simulink model "DF001A_FltInj"  (R2013b)
settings: Solver=FixedStepDiscrete  StartTime=0.0  StopTime=1  FixedStep=.002  RelTol=1e-3
values from neighbouring files (symbols this model uses):
  ARCHGLBPRM_180OVERPI_ULS_F32 = DataDict.Constant    [DF001A_FltInj_DataDict.m]
  ARCHGLBPRM_2PI_ULS_F32 = DataDict.Constant    [DF001A_FltInj_DataDict.m]
  FLOATTOU0P16MULT_ULS_F32 = DataDict.Constant    [DF001A_FltInj_DataDict.m]
  TICNVN_MILLISECPERCNT_F32 = DataDict.Constant    [DF001A_FltInj_DataDict.m]
libraries: simulink x6, NxtrLim x2, NxtrAbslt x1, NxtrMath x1, FixdToFloat x1
(part 2 of 2)

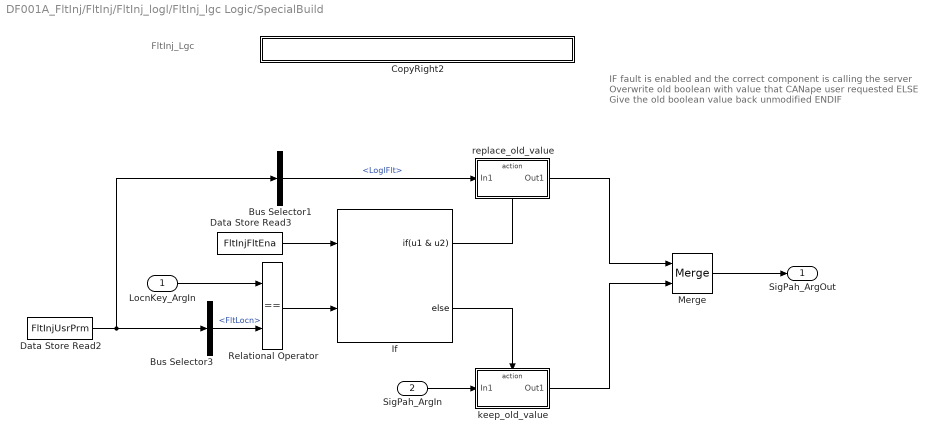
== system DF001A_FltInj/FltInj/FltInj_logl/FltInj_lgc Logic/SpecialBuild ==
  note: IF  fault is enabled and the correct component is calling the server
      |     Overwrite old boolean with value that CANape user requested
      | ELSE
      |     Give the old boolean value back unmodified
      | ENDIF
  note: FltInj_Lgc
  LocnKey_ArgIn : Inport  RequirementInfo={} %GIDa_ad100357_96bd_46c3_ad57_bbc8d7f94a2d
  SigPah_ArgIn : Inport  RequirementInfo={} %GIDa_10444aa2_7cb6_4718_9162_edb39688d745  Port=2
  Bus Selector1 : BusSelector  OutputSignals=LoglFlt
  Bus Selector3 : BusSelector  OutputSignals=FltLocn
  CopyRight2 : Subsystem  Description=|  mask(Copyright Information){none=on}
      | Copyright info block.                                               
      |                                                                     
      | Place copyright information at the top of every subsystem in design.
      mask prompts: none "No parameters"
      mask help: Place copyright information at the top of every subsystem in design.
      mask Display:
      | NxtrConf = 'Nexteer Confidential';
      | 
      | sys = bdroot; %handle for the current model ("system")
      | first = get_param(sys,'Created');
      | if(isempty(first))
      |     first = datestr(now,'yyyy');
      | else
      |     first = first(end-3:end);  %year is last four digits
      | end
      | 
      | last = get_param(sys,'LastModifiedDate');
      | if isempty(last)
      |     last = datestr(now,'yyyy');
      | else
      |     last = last(end-3:end);
      | end
      | 
      | if strcmp(first,last)
      |     fprintf('%s -- Copyright %s Nexteer',NxtrConf,first)
      | else
      |     fprintf('%s -- %s%s- %s Nexteer',NxtrConf,char(169),first,last)
      | end
  Data Store Read2 : DataStoreRead  DataStoreName=FltInjUsrPrm
  Data Store Read3 : DataStoreRead  DataStoreName=FltInjFltEna
  If : If  NumInputs=2  IfExpression=u1 & u2
  Merge : Merge
  Relational Operator : RelationalOperator  Operator===
  keep_old_value : Subsystem  TreatAsAtomicUnit=on
  replace_old_value : Subsystem  TreatAsAtomicUnit=on
  SigPah_ArgOut : Outport
  wires:
  Merge/1 -> SigPah_ArgOut/1
  Data Store Read2/1 -> Bus Selector1/1, Bus Selector3/1
  Bus Selector3/1 -> Relational Operator/2  "<FltLocn>"
  Data Store Read3/1 -> If/1
  If/2 -> keep_old_value/Action
  SigPah_ArgIn/1 -> keep_old_value/1(In1)
  If/1 -> replace_old_value/Action
  Bus Selector1/1 -> replace_old_value/1(In1)  "<LoglFlt>"
  replace_old_value/1(Out1) -> Merge/1
  keep_old_value/1(Out1) -> Merge/2
  LocnKey_ArgIn/1 -> Relational Operator/1
  Relational Operator/1 -> If/2

== system DF001A_FltInj/FltInj/FltInj_u08/ FltInj_u08 Logic/CopyRight2 ==

== system DF001A_FltInj/FltInj/FltInj_u08/ FltInj_u08 Logic/ProductionBuild ==
  PahGain : Inport  RequirementInfo={} %GIDa_51bd046f_2a11_4d13_8e15_9933e1cae419
  PahOffs : Inport  RequirementInfo={} %GIDa_330d29f2_2b4a_4e4f_bf37_c420c78ff4a3  Port=2
  SigPah_ArgIn : Inport  RequirementInfo={} %GIDa_d2bf9c39_34e5_4216_be9c_24ef8b9d2167  Port=3
  LocnKey_ArgIn : Inport  RequirementInfo={} %GIDa_1f9563e9_8098_41f5_bebe_21ae10e2094c  Port=4
  CopyRight2 : Subsystem  Description=|  mask(Copyright Information){none=on}
      | Copyright info block.                                               
      |                                                                     
      | Place copyright information at the top of every subsystem in design.
      mask prompts: none "No parameters"
      mask help: Place copyright information at the top of every subsystem in design.
      mask Display:
      | NxtrConf = 'Nexteer Confidential';
      | 
      | sys = bdroot; %handle for the current model ("system")
      | first = get_param(sys,'Created');
      | if(isempty(first))
      |     first = datestr(now,'yyyy');
      | else
      |     first = first(end-3:end);  %year is last four digits
      | end
      | 
      | last = get_param(sys,'LastModifiedDate');
      | if isempty(last)
      |     last = datestr(now,'yyyy');
      | else
      |     last = last(end-3:end);
      | end
      | 
      | if strcmp(first,last)
      |     fprintf('%s -- Copyright %s Nexteer',NxtrConf,first)
      | else
      |     fprintf('%s -- %s%s- %s Nexteer',NxtrConf,char(169),first,last)
      | end
  Ground : Ground
  Terminator{,1,3..4} (4 alike) : Terminator
  SigPah_ArgOut : Outport
  wires:
  PahGain/1 -> Terminator/1
  PahOffs/1 -> Terminator1/1
  SigPah_ArgIn/1 -> Terminator3/1
  LocnKey_ArgIn/1 -> Terminator4/1
  Ground/1 -> SigPah_ArgOut/1

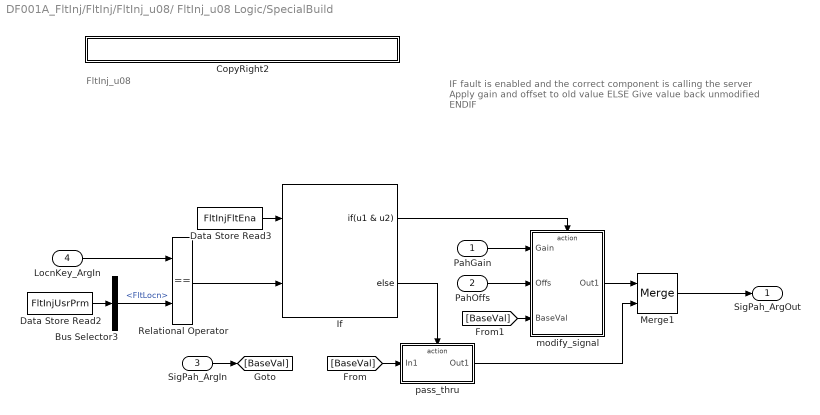
== system DF001A_FltInj/FltInj/FltInj_u08/ FltInj_u08 Logic/SpecialBuild ==
  note: IF  fault is enabled and the correct component is calling the server
      |     Apply gain and offset to old value
      | ELSE
      |     Give value back unmodified
      | ENDIF
  note: FltInj_u08
  PahGain : Inport  RequirementInfo={} %GIDa_09a7909a_afc0_4e82_9d6d_fea4d1cc2d4b
  PahOffs : Inport  RequirementInfo={} %GIDa_efc83883_c02f_44d9_abc4_963e9b64a895  Port=2
  SigPah_ArgIn : Inport  RequirementInfo={} %GIDa_0379ccaf_df52_493d_9083_89fc430c3f6f  Port=3
  LocnKey_ArgIn : Inport  RequirementInfo={} %GIDa_ad28a2fa_1a08_4c28_ae0d_7670c33a321e  Port=4
  Bus Selector3 : BusSelector  OutputSignals=FltLocn
  CopyRight2 : Subsystem  Description=|  mask(Copyright Information){none=on}
      | Copyright info block.                                               
      |                                                                     
      | Place copyright information at the top of every subsystem in design.
      mask prompts: none "No parameters"
      mask help: Place copyright information at the top of every subsystem in design.
      mask Display:
      | NxtrConf = 'Nexteer Confidential';
      | 
      | sys = bdroot; %handle for the current model ("system")
      | first = get_param(sys,'Created');
      | if(isempty(first))
      |     first = datestr(now,'yyyy');
      | else
      |     first = first(end-3:end);  %year is last four digits
      | end
      | 
      | last = get_param(sys,'LastModifiedDate');
      | if isempty(last)
      |     last = datestr(now,'yyyy');
      | else
      |     last = last(end-3:end);
      | end
      | 
      | if strcmp(first,last)
      |     fprintf('%s -- Copyright %s Nexteer',NxtrConf,first)
      | else
      |     fprintf('%s -- %s%s- %s Nexteer',NxtrConf,char(169),first,last)
      | end
  Data Store Read2 : DataStoreRead  DataStoreName=FltInjUsrPrm
  Data Store Read3 : DataStoreRead  DataStoreName=FltInjFltEna
  If : If  NumInputs=2  IfExpression=u1 & u2
  Merge1 : Merge
  Relational Operator : RelationalOperator  Operator===
  modify_signal : Subsystem  TreatAsAtomicUnit=on
  pass_thru : Subsystem  TreatAsAtomicUnit=on
  SigPah_ArgOut : Outport
  wires:
  Merge1/1 -> SigPah_ArgOut/1
  Data Store Read2/1 -> Bus Selector3/1
  PahGain/1 -> modify_signal/1(Gain)
  PahOffs/1 -> modify_signal/2(Offs)
  SigPah_ArgIn/1 -> [BaseVal]
  [BaseVal] -> pass_thru/1(In1)
  [BaseVal] -> modify_signal/3(BaseVal)
  If/1 -> modify_signal/Action
  If/2 -> pass_thru/Action
  modify_signal/1(Out1) -> Merge1/1
  pass_thru/1(Out1) -> Merge1/2
  Data Store Read3/1 -> If/1
  LocnKey_ArgIn/1 -> Relational Operator/1
  Bus Selector3/1 -> Relational Operator/2  "<FltLocn>"
  Relational Operator/1 -> If/2

== system DF001A_FltInj/FltInj/FltInj_u0p16/ FltInj_u0p16 Logic/CopyRight2 ==

== system DF001A_FltInj/FltInj/FltInj_u0p16/ FltInj_u0p16 Logic/ProductionBuild ==
  PahGain : Inport  RequirementInfo={} %GIDa_eb805554_5c38_478f_81b6_c594c852bef9
  PahOffs : Inport  RequirementInfo={} %GIDa_2ac31bbb_54e0_4ffb_a0b3_b3ade17ad800  Port=2
  SigPah_ArgIn : Inport  RequirementInfo={} %GIDa_203803f9_2924_4c5e_ad43_932bc0cde752  Port=3
  LocnKey_ArgIn : Inport  RequirementInfo={} %GIDa_37dd283f_5a7e_460f_b3ed_c0b52d76c8cf  Port=4
  CopyRight2 : Subsystem  Description=|  mask(Copyright Information){none=on}
      | Copyright info block.                                               
      |                                                                     
      | Place copyright information at the top of every subsystem in design.
      mask prompts: none "No parameters"
      mask help: Place copyright information at the top of every subsystem in design.
      mask Display:
      | NxtrConf = 'Nexteer Confidential';
      | 
      | sys = bdroot; %handle for the current model ("system")
      | first = get_param(sys,'Created');
      | if(isempty(first))
      |     first = datestr(now,'yyyy');
      | else
      |     first = first(end-3:end);  %year is last four digits
      | end
      | 
      | last = get_param(sys,'LastModifiedDate');
      | if isempty(last)
      |     last = datestr(now,'yyyy');
      | else
      |     last = last(end-3:end);
      | end
      | 
      | if strcmp(first,last)
      |     fprintf('%s -- Copyright %s Nexteer',NxtrConf,first)
      | else
      |     fprintf('%s -- %s%s- %s Nexteer',NxtrConf,char(169),first,last)
      | end
  Ground : Ground
  Terminator{,1,3..4} (4 alike) : Terminator
  SigPah_ArgOut : Outport
  wires:
  PahGain/1 -> Terminator/1
  PahOffs/1 -> Terminator1/1
  SigPah_ArgIn/1 -> Terminator3/1
  LocnKey_ArgIn/1 -> Terminator4/1
  Ground/1 -> SigPah_ArgOut/1

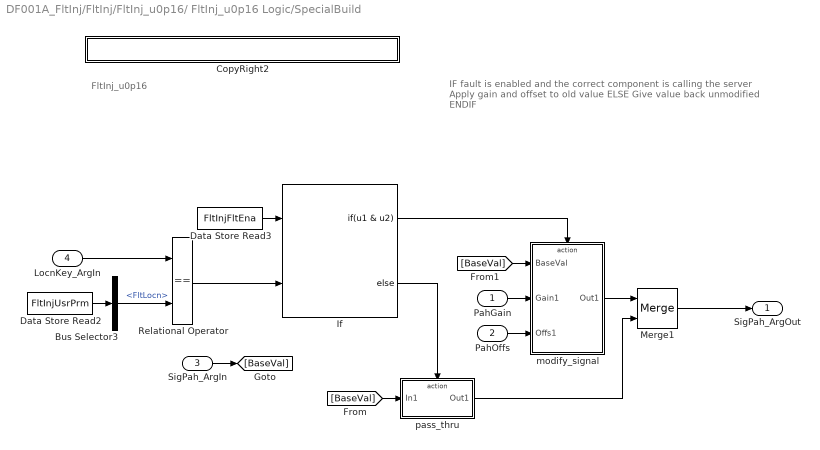
== system DF001A_FltInj/FltInj/FltInj_u0p16/ FltInj_u0p16 Logic/SpecialBuild ==
  note: IF  fault is enabled and the correct component is calling the server
      |     Apply gain and offset to old value
      | ELSE
      |     Give value back unmodified
      | ENDIF
  note: FltInj_u0p16
  PahGain : Inport  RequirementInfo={} %GIDa_9cb9172d_1f40_48e9_9430_512b7351e9fb
  PahOffs : Inport  RequirementInfo={} %GIDa_58d15e15_2c2f_4950_b5d5_3bf1f2651c55  Port=2
  SigPah_ArgIn : Inport  RequirementInfo={} %GIDa_1746ca05_6cb0_4872_9af5_1ff0a7839794  Port=3
  LocnKey_ArgIn : Inport  RequirementInfo={} %GIDa_14ac42b9_6095_4490_9fdf_0b61c79c8927  Port=4
  Bus Selector3 : BusSelector  OutputSignals=FltLocn
  CopyRight2 : Subsystem  Description=|  mask(Copyright Information){none=on}
      | Copyright info block.                                               
      |                                                                     
      | Place copyright information at the top of every subsystem in design.
      mask prompts: none "No parameters"
      mask help: Place copyright information at the top of every subsystem in design.
      mask Display:
      | NxtrConf = 'Nexteer Confidential';
      | 
      | sys = bdroot; %handle for the current model ("system")
      | first = get_param(sys,'Created');
      | if(isempty(first))
      |     first = datestr(now,'yyyy');
      | else
      |     first = first(end-3:end);  %year is last four digits
      | end
      | 
      | last = get_param(sys,'LastModifiedDate');
      | if isempty(last)
      |     last = datestr(now,'yyyy');
      | else
      |     last = last(end-3:end);
      | end
      | 
      | if strcmp(first,last)
      |     fprintf('%s -- Copyright %s Nexteer',NxtrConf,first)
      | else
      |     fprintf('%s -- %s%s- %s Nexteer',NxtrConf,char(169),first,last)
      | end
  Data Store Read2 : DataStoreRead  DataStoreName=FltInjUsrPrm
  Data Store Read3 : DataStoreRead  DataStoreName=FltInjFltEna
  If : If  NumInputs=2  IfExpression=u1 & u2
  Merge1 : Merge
  Relational Operator : RelationalOperator  Operator===
  modify_signal : Subsystem  TreatAsAtomicUnit=on
  pass_thru : Subsystem  TreatAsAtomicUnit=on
  SigPah_ArgOut : Outport
  wires:
  Merge1/1 -> SigPah_ArgOut/1
  Data Store Read2/1 -> Bus Selector3/1
  SigPah_ArgIn/1 -> [BaseVal]
  [BaseVal] -> pass_thru/1(In1)
  [BaseVal] -> modify_signal/1(BaseVal)
  If/1 -> modify_signal/Action
  If/2 -> pass_thru/Action
  modify_signal/1(Out1) -> Merge1/1
  pass_thru/1(Out1) -> Merge1/2
  Data Store Read3/1 -> If/1
  LocnKey_ArgIn/1 -> Relational Operator/1
  Bus Selector3/1 -> Relational Operator/2  "<FltLocn>"
  Relational Operator/1 -> If/2
  PahGain/1 -> modify_signal/2(Gain1)
  PahOffs/1 -> modify_signal/3(Offs1)

== system DF001A_FltInj/FltInj/FltInjPer1/Per1 Logic/ProductionBuild/CopyRight2 ==

== system DF001A_FltInj/FltInj/FltInjPer1/Per1 Logic/SpecialBuild/Begin_FaultInj ==
  UsrPrm : Inport
  Action Port : ActionPort  ActionType=elseif
  Bus Selector3 : BusSelector  OutputSignals=FltGain,FltOffs
  Constant1 : Constant  Value=true  OutDataTypeStr=boolean
  CopyRight2 : Subsystem  Description=|  mask(Copyright Information){none=on}
      | Copyright info block.                                               
      |                                                                     
      | Place copyright information at the top of every subsystem in design.
      mask prompts: none "No parameters"
      mask help: Place copyright information at the top of every subsystem in design.
      mask Display:
      | NxtrConf = 'Nexteer Confidential';
      | 
      | sys = bdroot; %handle for the current model ("system")
      | first = get_param(sys,'Created');
      | if(isempty(first))
      |     first = datestr(now,'yyyy');
      | else
      |     first = first(end-3:end);  %year is last four digits
      | end
      | 
      | last = get_param(sys,'LastModifiedDate');
      | if isempty(last)
      |     last = datestr(now,'yyyy');
      | else
      |     last = last(end-3:end);
      | end
      | 
      | if strcmp(first,last)
      |     fprintf('%s -- Copyright %s Nexteer',NxtrConf,first)
      | else
      |     fprintf('%s -- %s%s- %s Nexteer',NxtrConf,char(169),first,last)
      | end
  Data Store Write7 : DataStoreWrite  DataStoreName=FltInjRefTmr
  GetRefTmr100MicroSec32bit : Subsystem
  Signal Conversion : SignalConversion
  Signal Conversion1 : SignalConversion
  ArbdFltEna : Outport
  ArbdGain : Outport  Port=2
  ArbdOffs : Outport  Port=3
  wires:
  GetRefTmr100MicroSec32bit/1(RefTmr) -> Data Store Write7/1
  Constant1/1 -> ArbdFltEna/1  "ArbdFltEna"
  Bus Selector3/1 -> Signal Conversion/1  "<FltGain>"
  UsrPrm/1 -> Bus Selector3/1
  Signal Conversion/1 -> ArbdGain/1  "ArbdGain"
  Bus Selector3/2 -> Signal Conversion1/1  "<FltOffs>"
  Signal Conversion1/1 -> ArbdOffs/1  "ArbdOffs"

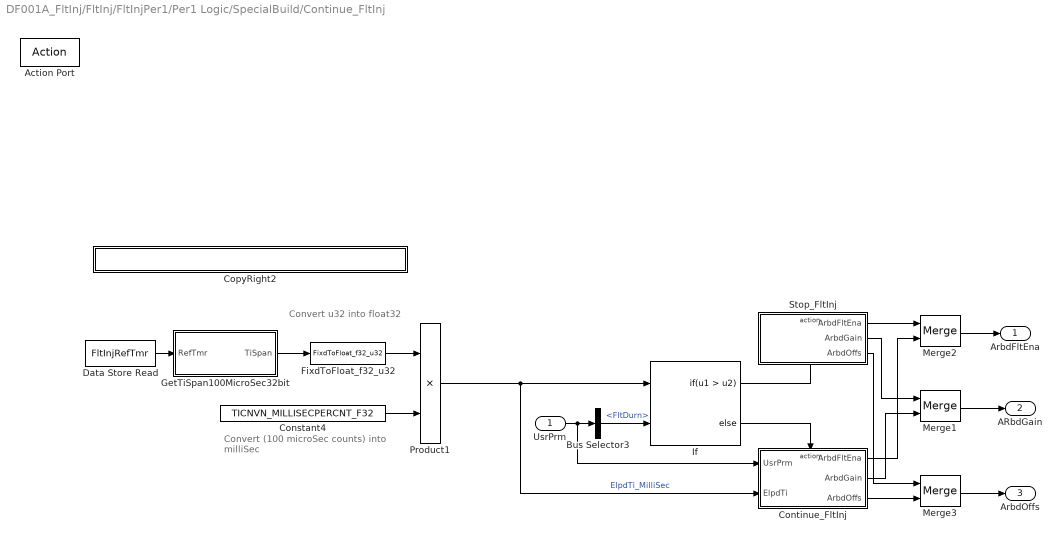
== system DF001A_FltInj/FltInj/FltInjPer1/Per1 Logic/SpecialBuild/Continue_FltInj ==
  note: Convert u32 into float32
  note: Convert (100 microSec counts)
      | into  milliSec
  UsrPrm : Inport
  Action Port : ActionPort  ActionType=else
  Bus Selector3 : BusSelector  OutputSignals=FltDurn
  Constant4 : Constant  Value=TICNVN_MILLISECPERCNT_F32
  Continue_FltInj : Subsystem  TreatAsAtomicUnit=on
  CopyRight2 : Subsystem  Description=|  mask(Copyright Information){none=on}
      | Copyright info block.                                               
      |                                                                     
      | Place copyright information at the top of every subsystem in design.
      mask prompts: none "No parameters"
      mask help: Place copyright information at the top of every subsystem in design.
      mask Display:
      | NxtrConf = 'Nexteer Confidential';
      | 
      | sys = bdroot; %handle for the current model ("system")
      | first = get_param(sys,'Created');
      | if(isempty(first))
      |     first = datestr(now,'yyyy');
      | else
      |     first = first(end-3:end);  %year is last four digits
      | end
      | 
      | last = get_param(sys,'LastModifiedDate');
      | if isempty(last)
      |     last = datestr(now,'yyyy');
      | else
      |     last = last(end-3:end);
      | end
      | 
      | if strcmp(first,last)
      |     fprintf('%s -- Copyright %s Nexteer',NxtrConf,first)
      | else
      |     fprintf('%s -- %s%s- %s Nexteer',NxtrConf,char(169),first,last)
      | end
  Data Store Read : DataStoreRead  DataStoreName=FltInjRefTmr
  FixdToFloat_f32_u32 : FixdToFloat/FixdToFloat_f32_u32  Param1=0
  GetTiSpan100MicroSec32bit : Subsystem
  If : If  NumInputs=2  IfExpression=u1 > u2
  Merge1 : Merge
  Merge2 : Merge
  Merge3 : Merge
  Product1 : Product  RndMeth=Zero
  Stop_FltInj : Subsystem  TreatAsAtomicUnit=on
  ArbdFltEna : Outport
  ARbdGain : Outport  Port=2
  ArbdOffs : Outport  Port=3
  wires:
  Data Store Read/1 -> GetTiSpan100MicroSec32bit/1(RefTmr)
  Constant4/1 -> Product1/2
  GetTiSpan100MicroSec32bit/1(TiSpan) -> FixdToFloat_f32_u32/1
  FixdToFloat_f32_u32/1 -> Product1/1
  Bus Selector3/1 -> If/2  "<FltDurn>"
  If/1 -> Stop_FltInj/Action
  If/2 -> Continue_FltInj/Action
  Merge2/1 -> ArbdFltEna/1
  Stop_FltInj/1(ArbdFltEna) -> Merge2/1
  Continue_FltInj/1(ArbdFltEna) -> Merge2/2
  Product1/1 -> Continue_FltInj/2(ElpdTi), If/1  "ElpdTi_MilliSec"
  UsrPrm/1 -> Continue_FltInj/1(UsrPrm), Bus Selector3/1
  Stop_FltInj/2(ArbdGain) -> Merge1/1
  Stop_FltInj/3(ArbdOffs) -> Merge3/1
  Continue_FltInj/2(ArbdGain) -> Merge1/2
  Continue_FltInj/3(ArbdOffs) -> Merge3/2
  Merge1/1 -> ARbdGain/1
  Merge3/1 -> ArbdOffs/1

== system DF001A_FltInj/FltInj/FltInjPer1/Per1 Logic/SpecialBuild/CopyRight2 ==

== system DF001A_FltInj/FltInj/FltInjPer1/Per1 Logic/SpecialBuild/Disable_FltInj ==
  Action Port : ActionPort  ActionType=then
  Constant2 : Constant  Value=false  OutDataTypeStr=boolean
  Constant3 : Constant  OutDataTypeStr=single
  Constant4 : Constant  Value=0  OutDataTypeStr=single
  CopyRight2 : Subsystem  Description=|  mask(Copyright Information){none=on}
      | Copyright info block.                                               
      |                                                                     
      | Place copyright information at the top of every subsystem in design.
      mask prompts: none "No parameters"
      mask help: Place copyright information at the top of every subsystem in design.
      mask Display:
      | NxtrConf = 'Nexteer Confidential';
      | 
      | sys = bdroot; %handle for the current model ("system")
      | first = get_param(sys,'Created');
      | if(isempty(first))
      |     first = datestr(now,'yyyy');
      | else
      |     first = first(end-3:end);  %year is last four digits
      | end
      | 
      | last = get_param(sys,'LastModifiedDate');
      | if isempty(last)
      |     last = datestr(now,'yyyy');
      | else
      |     last = last(end-3:end);
      | end
      | 
      | if strcmp(first,last)
      |     fprintf('%s -- Copyright %s Nexteer',NxtrConf,first)
      | else
      |     fprintf('%s -- %s%s- %s Nexteer',NxtrConf,char(169),first,last)
      | end
  ArbdFltEna : Outport
  ArbdGain : Outport  Port=2
  ArbdOffs : Outport  Port=3
  wires:
  Constant2/1 -> ArbdFltEna/1  "ArbdFltEna"
  Constant3/1 -> ArbdGain/1  "ArbdGain"
  Constant4/1 -> ArbdOffs/1  "ArbdOffs"

== system DF001A_FltInj/FltInj/FltInj_f32/ FltInj_f32 Logic/ProductionBuild/CopyRight2 ==

== system DF001A_FltInj/FltInj/FltInj_f32/ FltInj_f32 Logic/SpecialBuild/CopyRight2 ==

== system DF001A_FltInj/FltInj/FltInj_f32/ FltInj_f32 Logic/SpecialBuild/modify_signal ==
  Gain : Inport
  Offs : Inport  Port=2
  BaseVal : Inport  Port=3
  Action Port : ActionPort  ActionType=then
  Add : Sum
  CopyRight2 : Subsystem  Description=|  mask(Copyright Information){none=on}
      | Copyright info block.                                               
      |                                                                     
      | Place copyright information at the top of every subsystem in design.
      mask prompts: none "No parameters"
      mask help: Place copyright information at the top of every subsystem in design.
      mask Display:
      | NxtrConf = 'Nexteer Confidential';
      | 
      | sys = bdroot; %handle for the current model ("system")
      | first = get_param(sys,'Created');
      | if(isempty(first))
      |     first = datestr(now,'yyyy');
      | else
      |     first = first(end-3:end);  %year is last four digits
      | end
      | 
      | last = get_param(sys,'LastModifiedDate');
      | if isempty(last)
      |     last = datestr(now,'yyyy');
      | else
      |     last = last(end-3:end);
      | end
      | 
      | if strcmp(first,last)
      |     fprintf('%s -- Copyright %s Nexteer',NxtrConf,first)
      | else
      |     fprintf('%s -- %s%s- %s Nexteer',NxtrConf,char(169),first,last)
      | end
  Product : Product
  Out1 : Outport
  wires:
  Add/1 -> Out1/1
  BaseVal/1 -> Product/1
  Gain/1 -> Product/2
  Product/1 -> Add/1
  Offs/1 -> Add/2

== system DF001A_FltInj/FltInj/FltInj_f32/ FltInj_f32 Logic/SpecialBuild/pass_thru ==
  In1 : Inport
  Action Port : ActionPort  ActionType=else
  CopyRight2 : Subsystem  Description=|  mask(Copyright Information){none=on}
      | Copyright info block.                                               
      |                                                                     
      | Place copyright information at the top of every subsystem in design.
      mask prompts: none "No parameters"
      mask help: Place copyright information at the top of every subsystem in design.
      mask Display:
      | NxtrConf = 'Nexteer Confidential';
      | 
      | sys = bdroot; %handle for the current model ("system")
      | first = get_param(sys,'Created');
      | if(isempty(first))
      |     first = datestr(now,'yyyy');
      | else
      |     first = first(end-3:end);  %year is last four digits
      | end
      | 
      | last = get_param(sys,'LastModifiedDate');
      | if isempty(last)
      |     last = datestr(now,'yyyy');
      | else
      |     last = last(end-3:end);
      | end
      | 
      | if strcmp(first,last)
      |     fprintf('%s -- Copyright %s Nexteer',NxtrConf,first)
      | else
      |     fprintf('%s -- %s%s- %s Nexteer',NxtrConf,char(169),first,last)
      | end
  Out1 : Outport
  wires:
  In1/1 -> Out1/1

== system DF001A_FltInj/FltInj/FltInj_logl/FltInj_lgc Logic/ProductionBuild/CopyRight2 ==

== system DF001A_FltInj/FltInj/FltInj_logl/FltInj_lgc Logic/SpecialBuild/CopyRight2 ==

== system DF001A_FltInj/FltInj/FltInj_logl/FltInj_lgc Logic/SpecialBuild/keep_old_value ==
  In1 : Inport
  Action Port : ActionPort  ActionType=else
  CopyRight2 : Subsystem  Description=|  mask(Copyright Information){none=on}
      | Copyright info block.                                               
      |                                                                     
      | Place copyright information at the top of every subsystem in design.
      mask prompts: none "No parameters"
      mask help: Place copyright information at the top of every subsystem in design.
      mask Display:
      | NxtrConf = 'Nexteer Confidential';
      | 
      | sys = bdroot; %handle for the current model ("system")
      | first = get_param(sys,'Created');
      | if(isempty(first))
      |     first = datestr(now,'yyyy');
      | else
      |     first = first(end-3:end);  %year is last four digits
      | end
      | 
      | last = get_param(sys,'LastModifiedDate');
      | if isempty(last)
      |     last = datestr(now,'yyyy');
      | else
      |     last = last(end-3:end);
      | end
      | 
      | if strcmp(first,last)
      |     fprintf('%s -- Copyright %s Nexteer',NxtrConf,first)
      | else
      |     fprintf('%s -- %s%s- %s Nexteer',NxtrConf,char(169),first,last)
      | end
  Out1 : Outport
  wires:
  In1/1 -> Out1/1

== system DF001A_FltInj/FltInj/FltInj_logl/FltInj_lgc Logic/SpecialBuild/replace_old_value ==
  In1 : Inport
  Action Port : ActionPort  ActionType=then
  CopyRight2 : Subsystem  Description=|  mask(Copyright Information){none=on}
      | Copyright info block.                                               
      |                                                                     
      | Place copyright information at the top of every subsystem in design.
      mask prompts: none "No parameters"
      mask help: Place copyright information at the top of every subsystem in design.
      mask Display:
      | NxtrConf = 'Nexteer Confidential';
      | 
      | sys = bdroot; %handle for the current model ("system")
      | first = get_param(sys,'Created');
      | if(isempty(first))
      |     first = datestr(now,'yyyy');
      | else
      |     first = first(end-3:end);  %year is last four digits
      | end
      | 
      | last = get_param(sys,'LastModifiedDate');
      | if isempty(last)
      |     last = datestr(now,'yyyy');
      | else
      |     last = last(end-3:end);
      | end
      | 
      | if strcmp(first,last)
      |     fprintf('%s -- Copyright %s Nexteer',NxtrConf,first)
      | else
      |     fprintf('%s -- %s%s- %s Nexteer',NxtrConf,char(169),first,last)
      | end
  Out1 : Outport
  wires:
  In1/1 -> Out1/1

== system DF001A_FltInj/FltInj/FltInj_u08/ FltInj_u08 Logic/ProductionBuild/CopyRight2 ==

== system DF001A_FltInj/FltInj/FltInj_u08/ FltInj_u08 Logic/SpecialBuild/CopyRight2 ==

== system DF001A_FltInj/FltInj/FltInj_u08/ FltInj_u08 Logic/SpecialBuild/modify_signal ==
  note: FltInj_u08
  Gain : Inport
  Offs : Inport  Port=2
  BaseVal : Inport  Port=3
  Action Port : ActionPort  ActionType=then
  Add : Sum
  CopyRight2 : Subsystem  Description=|  mask(Copyright Information){none=on}
      | Copyright info block.                                               
      |                                                                     
      | Place copyright information at the top of every subsystem in design.
      mask prompts: none "No parameters"
      mask help: Place copyright information at the top of every subsystem in design.
      mask Display:
      | NxtrConf = 'Nexteer Confidential';
      | 
      | sys = bdroot; %handle for the current model ("system")
      | first = get_param(sys,'Created');
      | if(isempty(first))
      |     first = datestr(now,'yyyy');
      | else
      |     first = first(end-3:end);  %year is last four digits
      | end
      | 
      | last = get_param(sys,'LastModifiedDate');
      | if isempty(last)
      |     last = datestr(now,'yyyy');
      | else
      |     last = last(end-3:end);
      | end
      | 
      | if strcmp(first,last)
      |     fprintf('%s -- Copyright %s Nexteer',NxtrConf,first)
      | else
      |     fprintf('%s -- %s%s- %s Nexteer',NxtrConf,char(169),first,last)
      | end
  Data Type Conversion : DataTypeConversion  OutDataTypeStr=single
  Data Type Conversion1 : DataTypeConversion  OutDataTypeStr=uint8
  LimStat_f32 : NxtrLim/LimStat_f32  LoLim=0  HiLim=UINT8MAX_ULS_F32
      settings: AttributesFormatString=|
      | Low Limit: %<LoLim>
      | High Limit:%<HiLim>
  Product : Product
  Out1 : Outport
  wires:
  Add/1 -> LimStat_f32/1
  BaseVal/1 -> Data Type Conversion/1
  Gain/1 -> Product/2
  Product/1 -> Add/1
  Offs/1 -> Add/2
  Data Type Conversion/1 -> Product/1
  Data Type Conversion1/1 -> Out1/1
  LimStat_f32/1 -> Data Type Conversion1/1

== system DF001A_FltInj/FltInj/FltInj_u08/ FltInj_u08 Logic/SpecialBuild/pass_thru ==
  In1 : Inport
  Action Port : ActionPort  ActionType=else
  CopyRight2 : Subsystem  Description=|  mask(Copyright Information){none=on}
      | Copyright info block.                                               
      |                                                                     
      | Place copyright information at the top of every subsystem in design.
      mask prompts: none "No parameters"
      mask help: Place copyright information at the top of every subsystem in design.
      mask Display:
      | NxtrConf = 'Nexteer Confidential';
      | 
      | sys = bdroot; %handle for the current model ("system")
      | first = get_param(sys,'Created');
      | if(isempty(first))
      |     first = datestr(now,'yyyy');
      | else
      |     first = first(end-3:end);  %year is last four digits
      | end
      | 
      | last = get_param(sys,'LastModifiedDate');
      | if isempty(last)
      |     last = datestr(now,'yyyy');
      | else
      |     last = last(end-3:end);
      | end
      | 
      | if strcmp(first,last)
      |     fprintf('%s -- Copyright %s Nexteer',NxtrConf,first)
      | else
      |     fprintf('%s -- %s%s- %s Nexteer',NxtrConf,char(169),first,last)
      | end
  Out1 : Outport
  wires:
  In1/1 -> Out1/1

== system DF001A_FltInj/FltInj/FltInj_u0p16/ FltInj_u0p16 Logic/ProductionBuild/CopyRight2 ==

== system DF001A_FltInj/FltInj/FltInj_u0p16/ FltInj_u0p16 Logic/SpecialBuild/CopyRight2 ==

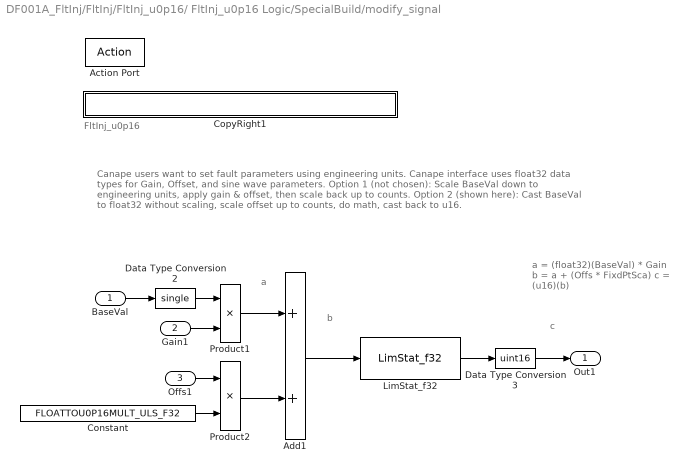
== system DF001A_FltInj/FltInj/FltInj_u0p16/ FltInj_u0p16 Logic/SpecialBuild/modify_signal ==
  note: FltInj_u0p16
  note: c
  note: b
  note: a
  note: Canape users want to set fault parameters using engineering units.
      | Canape interface uses float32 data types for Gain, Offset, and sine wave parameters.
      |
      | Option 1 (not chosen):  Scale BaseVal down to engineering units, apply gain & offset, then scale back up to counts.
      | Option 2 (shown here): Cast BaseVal to float32 without scaling, scale offset up to counts, do math, cast back to u16.
  note: a = (float32)(BaseVal) * Gain
      | b = a + (Offs * FixdPtSca)
      | c = (u16)(b)
  BaseVal : Inport
  Gain1 : Inport  Port=2
  Offs1 : Inport  Port=3
  Action Port : ActionPort  ActionType=then
  Add1 : Sum
  Constant : Constant  Value=FLOATTOU0P16MULT_ULS_F32
  CopyRight1 : Subsystem  Description=|  mask(Copyright Information){none=on}
      | Copyright info block.                                               
      |                                                                     
      | Place copyright information at the top of every subsystem in design.
      mask prompts: none "No parameters"
      mask help: Place copyright information at the top of every subsystem in design.
      mask Display:
      | NxtrConf = 'Nexteer Confidential';
      | 
      | sys = bdroot; %handle for the current model ("system")
      | first = get_param(sys,'Created');
      | if(isempty(first))
      |     first = datestr(now,'yyyy');
      | else
      |     first = first(end-3:end);  %year is last four digits
      | end
      | 
      | last = get_param(sys,'LastModifiedDate');
      | if isempty(last)
      |     last = datestr(now,'yyyy');
      | else
      |     last = last(end-3:end);
      | end
      | 
      | if strcmp(first,last)
      |     fprintf('%s -- Copyright %s Nexteer',NxtrConf,first)
      | else
      |     fprintf('%s -- %s%s- %s Nexteer',NxtrConf,char(169),first,last)
      | end
  Data Type Conversion2 : DataTypeConversion  OutDataTypeStr=single
  Data Type Conversion3 : DataTypeConversion  OutDataTypeStr=uint16
  LimStat_f32 : NxtrLim/LimStat_f32  LoLim=0  HiLim=UINT16MAX_ULS_F32
      settings: AttributesFormatString=|
      | Low Limit: %<LoLim>
      | High Limit:%<HiLim>
  Product1 : Product
  Product2 : Product
  Out1 : Outport
  wires:
  Gain1/1 -> Product1/2
  Product1/1 -> Add1/1
  Data Type Conversion2/1 -> Product1/1
  Add1/1 -> LimStat_f32/1
  Offs1/1 -> Product2/1
  Constant/1 -> Product2/2
  Product2/1 -> Add1/2
  LimStat_f32/1 -> Data Type Conversion3/1
  BaseVal/1 -> Data Type Conversion2/1
  Data Type Conversion3/1 -> Out1/1

== system DF001A_FltInj/FltInj/FltInj_u0p16/ FltInj_u0p16 Logic/SpecialBuild/pass_thru ==
  In1 : Inport
  Action Port : ActionPort  ActionType=else
  CopyRight2 : Subsystem  Description=|  mask(Copyright Information){none=on}
      | Copyright info block.                                               
      |                                                                     
      | Place copyright information at the top of every subsystem in design.
      mask prompts: none "No parameters"
      mask help: Place copyright information at the top of every subsystem in design.
      mask Display:
      | NxtrConf = 'Nexteer Confidential';
      | 
      | sys = bdroot; %handle for the current model ("system")
      | first = get_param(sys,'Created');
      | if(isempty(first))
      |     first = datestr(now,'yyyy');
      | else
      |     first = first(end-3:end);  %year is last four digits
      | end
      | 
      | last = get_param(sys,'LastModifiedDate');
      | if isempty(last)
      |     last = datestr(now,'yyyy');
      | else
      |     last = last(end-3:end);
      | end
      | 
      | if strcmp(first,last)
      |     fprintf('%s -- Copyright %s Nexteer',NxtrConf,first)
      | else
      |     fprintf('%s -- %s%s- %s Nexteer',NxtrConf,char(169),first,last)
      | end
  Out1 : Outport
  wires:
  In1/1 -> Out1/1

== system DF001A_FltInj/FltInj/FltInjPer1/Per1 Logic/SpecialBuild/Begin_FaultInj/CopyRight2 ==

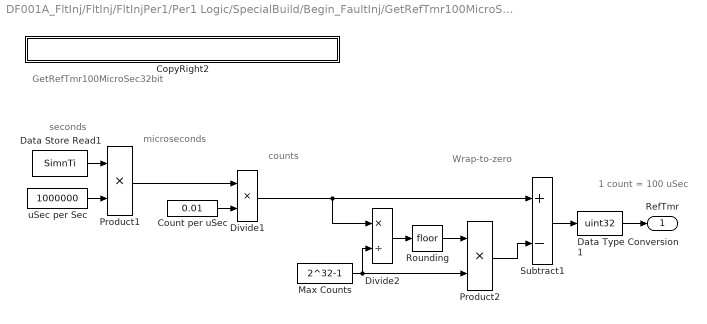
== system DF001A_FltInj/FltInj/FltInjPer1/Per1 Logic/SpecialBuild/Begin_FaultInj/GetRefTmr100MicroSec32bit ==
  note: GetRefTmr100MicroSec32bit
  note: Wrap-to-zero
  note: counts
  note: microseconds
  note: seconds
  note: 1 count = 100 uSec
  CopyRight2 : Subsystem  Description=|  mask(Copyright Information){none=on}
      | Copyright info block.                                               
      |                                                                     
      | Place copyright information at the top of every subsystem in design.
      mask prompts: none "No parameters"
      mask help: Place copyright information at the top of every subsystem in design.
      mask Display:
      | NxtrConf = 'Nexteer Confidential';
      | 
      | sys = bdroot; %handle for the current model ("system")
      | first = get_param(sys,'Created');
      | if(isempty(first))
      |     first = datestr(now,'yyyy');
      | else
      |     first = first(end-3:end);  %year is last four digits
      | end
      | 
      | last = get_param(sys,'LastModifiedDate');
      | if isempty(last)
      |     last = datestr(now,'yyyy');
      | else
      |     last = last(end-3:end);
      | end
      | 
      | if strcmp(first,last)
      |     fprintf('%s -- Copyright %s Nexteer',NxtrConf,first)
      | else
      |     fprintf('%s -- %s%s- %s Nexteer',NxtrConf,char(169),first,last)
      | end
  Count per uSec : Constant  Value=0.01
  Data Store Read1 : DataStoreRead  DataStoreName=SimnTi
  Data Type Conversion1 : DataTypeConversion  OutDataTypeStr=uint32
  Divide1 : Product  Inputs=**
  Divide2 : Product  Inputs=*/
  Max Counts : Constant  Value=2^32-1
  Product1 : Product
  Product2 : Product
  Rounding : Rounding
  Subtract1 : Sum  Inputs=+-
  uSec per Sec : Constant  Value=1000000
  RefTmr : Outport
  wires:
  Data Type Conversion1/1 -> RefTmr/1
  uSec per Sec/1 -> Product1/2
  Count per uSec/1 -> Divide1/2
  Data Store Read1/1 -> Product1/1
  Product1/1 -> Divide1/1
  Divide1/1 -> Subtract1/1, Divide2/1
  Max Counts/1 -> Product2/2, Divide2/2
  Divide2/1 -> Rounding/1
  Rounding/1 -> Product2/1
  Subtract1/1 -> Data Type Conversion1/1
  Product2/1 -> Subtract1/2

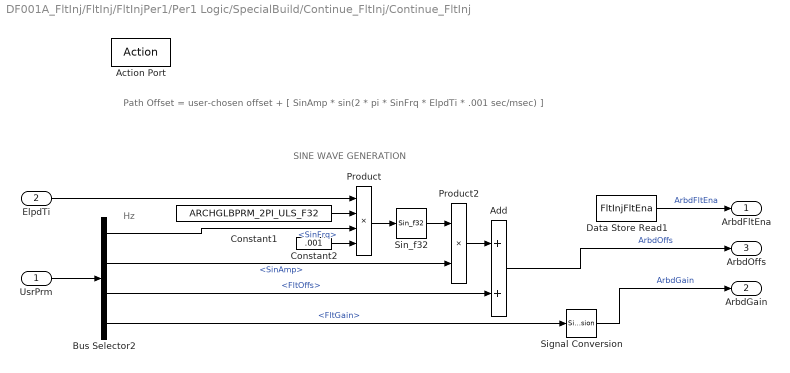
== system DF001A_FltInj/FltInj/FltInjPer1/Per1 Logic/SpecialBuild/Continue_FltInj/Continue_FltInj ==
  note: SINE WAVE GENERATION
  note: Hz
  note: Path Offset = user-chosen offset + [ SinAmp * sin(2 * pi * SinFrq * ElpdTi * .001 sec/msec) ]
  UsrPrm : Inport
  ElpdTi : Inport  Port=2
  Action Port : ActionPort  ActionType=else
  Add : Sum
  Bus Selector2 : BusSelector  OutputSignals=SinFrq,SinAmp,FltOffs,FltGain
  Constant1 : Constant  Value=ARCHGLBPRM_2PI_ULS_F32
  Constant2 : Constant  Value=.001
  Data Store Read1 : DataStoreRead  DataStoreName=FltInjFltEna
  Product : Product  Inputs=4
  Product2 : Product
  Signal Conversion : SignalConversion
  Sin_f32 : NxtrMath/Sin_f32  SFunctionSpec=single y1 = Sin_f32(single u1)
      settings: AttributesFormatString=%<MaskType>
  ArbdFltEna : Outport
  ArbdGain : Outport  Port=2
  ArbdOffs : Outport  Port=3
  wires:
  Data Store Read1/1 -> ArbdFltEna/1  "ArbdFltEna"
  Bus Selector2/1 -> Product/3  "<SinFrq>"
  Bus Selector2/2 -> Product2/2  "<SinAmp>"
  Product/1 -> Sin_f32/1
  Sin_f32/1 -> Product2/1
  Constant2/1 -> Product/4
  Constant1/1 -> Product/2
  UsrPrm/1 -> Bus Selector2/1
  Product2/1 -> Add/1
  Bus Selector2/3 -> Add/2  "<FltOffs>"
  Add/1 -> ArbdOffs/1  "ArbdOffs"
  Bus Selector2/4 -> Signal Conversion/1  "<FltGain>"
  Signal Conversion/1 -> ArbdGain/1  "ArbdGain"
  ElpdTi/1 -> Product/1

== system DF001A_FltInj/FltInj/FltInjPer1/Per1 Logic/SpecialBuild/Continue_FltInj/CopyRight2 ==

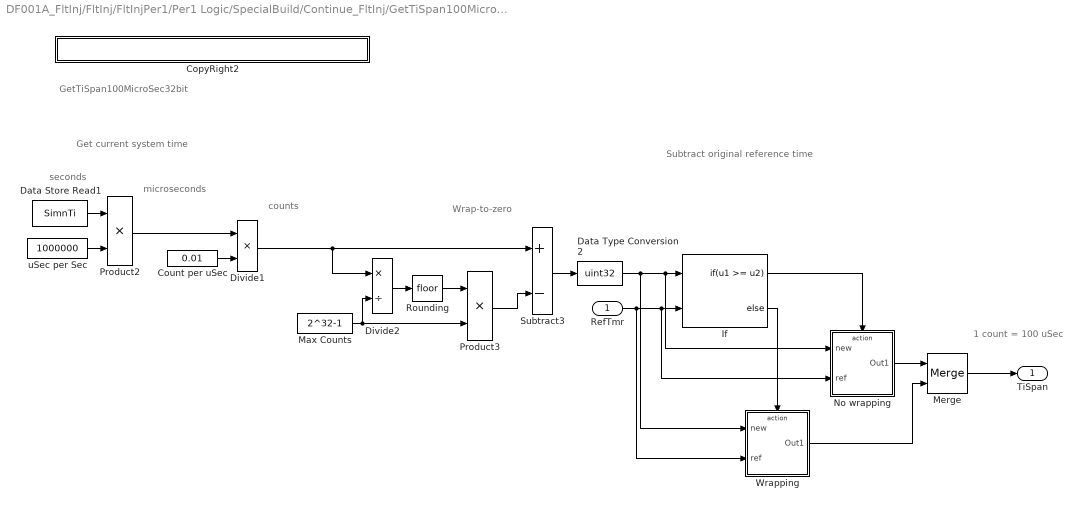
== system DF001A_FltInj/FltInj/FltInjPer1/Per1 Logic/SpecialBuild/Continue_FltInj/GetTiSpan100MicroSec32bit ==
  note: GetTiSpan100MicroSec32bit
  note: Get current system time
  note: 1 count = 100 uSec
  note: Wrap-to-zero
  note: counts
  note: microseconds
  note: seconds
  note: Subtract original reference time
  RefTmr : Inport
  CopyRight2 : Subsystem  Description=|  mask(Copyright Information){none=on}
      | Copyright info block.                                               
      |                                                                     
      | Place copyright information at the top of every subsystem in design.
      mask prompts: none "No parameters"
      mask help: Place copyright information at the top of every subsystem in design.
      mask Display:
      | NxtrConf = 'Nexteer Confidential';
      | 
      | sys = bdroot; %handle for the current model ("system")
      | first = get_param(sys,'Created');
      | if(isempty(first))
      |     first = datestr(now,'yyyy');
      | else
      |     first = first(end-3:end);  %year is last four digits
      | end
      | 
      | last = get_param(sys,'LastModifiedDate');
      | if isempty(last)
      |     last = datestr(now,'yyyy');
      | else
      |     last = last(end-3:end);
      | end
      | 
      | if strcmp(first,last)
      |     fprintf('%s -- Copyright %s Nexteer',NxtrConf,first)
      | else
      |     fprintf('%s -- %s%s- %s Nexteer',NxtrConf,char(169),first,last)
      | end
  Count per uSec : Constant  Value=0.01
  Data Store Read1 : DataStoreRead  DataStoreName=SimnTi
  Data Type Conversion2 : DataTypeConversion  OutDataTypeStr=uint32
  Divide1 : Product  Inputs=**
  Divide2 : Product  Inputs=*/
  If : If  NumInputs=2  IfExpression=u1 >= u2
  Max Counts : Constant  Value=2^32-1
  Merge : Merge
  No wrapping : Subsystem  TreatAsAtomicUnit=on
  Product2 : Product
  Product3 : Product
  Rounding : Rounding
  Subtract3 : Sum  Inputs=+-
  Wrapping : Subsystem  TreatAsAtomicUnit=on
  uSec per Sec : Constant  Value=1000000
  TiSpan : Outport
  wires:
  Data Type Conversion2/1 -> Wrapping/1(new), No wrapping/1(new), If/1
  RefTmr/1 -> Wrapping/2(ref), No wrapping/2(ref), If/2
  Merge/1 -> TiSpan/1
  uSec per Sec/1 -> Product2/2
  Count per uSec/1 -> Divide1/2
  Data Store Read1/1 -> Product2/1
  Product2/1 -> Divide1/1
  Divide1/1 -> Subtract3/1, Divide2/1
  Max Counts/1 -> Product3/2, Divide2/2
  Divide2/1 -> Rounding/1
  Rounding/1 -> Product3/1
  Subtract3/1 -> Data Type Conversion2/1
  Product3/1 -> Subtract3/2
  If/1 -> No wrapping/Action
  If/2 -> Wrapping/Action
  No wrapping/1(Out1) -> Merge/1
  Wrapping/1(Out1) -> Merge/2

== system DF001A_FltInj/FltInj/FltInjPer1/Per1 Logic/SpecialBuild/Continue_FltInj/Stop_FltInj ==
  note: Set CANape's value to false to ensure that the fault occurs only one time until CANape user manually re-enables it.
  Action Port : ActionPort  ActionType=then
  Constant1 : Constant  Value=false  OutDataTypeStr=boolean
  Constant2 : Constant  Value=false  OutDataTypeStr=boolean
  Constant3 : Constant  OutDataTypeStr=single
  Constant4 : Constant  Value=0  OutDataTypeStr=single
  Data Store Write : DataStoreWrite  DataStoreName=FltInjUsrPrm  DataStoreElements=FltInjUsrPrm.FltInjEna
  ArbdFltEna : Outport
  ArbdGain : Outport  Port=2
  ArbdOffs : Outport  Port=3
  wires:
  Constant2/1 -> ArbdFltEna/1  "ArbdFltEna"
  Constant3/1 -> ArbdGain/1  "ArbdGain"
  Constant4/1 -> ArbdOffs/1  "ArbdOffs"
  Constant1/1 -> Data Store Write/1

== system DF001A_FltInj/FltInj/FltInjPer1/Per1 Logic/SpecialBuild/Disable_FltInj/CopyRight2 ==

== system DF001A_FltInj/FltInj/FltInj_f32/ FltInj_f32 Logic/SpecialBuild/modify_signal/CopyRight2 ==

== system DF001A_FltInj/FltInj/FltInj_f32/ FltInj_f32 Logic/SpecialBuild/pass_thru/CopyRight2 ==

== system DF001A_FltInj/FltInj/FltInj_logl/FltInj_lgc Logic/SpecialBuild/keep_old_value/CopyRight2 ==

== system DF001A_FltInj/FltInj/FltInj_logl/FltInj_lgc Logic/SpecialBuild/replace_old_value/CopyRight2 ==

== system DF001A_FltInj/FltInj/FltInj_u08/ FltInj_u08 Logic/SpecialBuild/modify_signal/CopyRight2 ==

== system DF001A_FltInj/FltInj/FltInj_u08/ FltInj_u08 Logic/SpecialBuild/pass_thru/CopyRight2 ==

== system DF001A_FltInj/FltInj/FltInj_u0p16/ FltInj_u0p16 Logic/SpecialBuild/modify_signal/CopyRight1 ==

== system DF001A_FltInj/FltInj/FltInj_u0p16/ FltInj_u0p16 Logic/SpecialBuild/pass_thru/CopyRight2 ==

== system DF001A_FltInj/FltInj/FltInjPer1/Per1 Logic/SpecialBuild/Begin_FaultInj/GetRefTmr100MicroSec32bit/CopyRight2 ==

== system DF001A_FltInj/FltInj/FltInjPer1/Per1 Logic/SpecialBuild/Continue_FltInj/GetTiSpan100MicroSec32bit/CopyRight2 ==

== system DF001A_FltInj/FltInj/FltInjPer1/Per1 Logic/SpecialBuild/Continue_FltInj/GetTiSpan100MicroSec32bit/No wrapping ==
  new : Inport
  ref : Inport  Port=2
  Action Port : ActionPort  ActionType=then
  Subtract1 : Sum  Inputs=+-
  Out1 : Outport
  wires:
  Subtract1/1 -> Out1/1
  new/1 -> Subtract1/1
  ref/1 -> Subtract1/2

== system DF001A_FltInj/FltInj/FltInjPer1/Per1 Logic/SpecialBuild/Continue_FltInj/GetTiSpan100MicroSec32bit/Wrapping ==
  new : Inport
  ref : Inport  Port=2
  Action Port : ActionPort  ActionType=else
  Max Counts : Constant  Value=2^32-1  OutDataTypeStr=uint32
  Subtract1 : Sum  Inputs=+-+
  Out1 : Outport
  wires:
  Subtract1/1 -> Out1/1
  Max Counts/1 -> Subtract1/1
  ref/1 -> Subtract1/2
  new/1 -> Subtract1/3
